simulink model "modelo_completo"  (R2023b)
settings: Solver=VariableStepAuto  StartTime=0.0  StopTime=10.0  RelTol=1e-3
undefined symbols (not defined in the file): T_hm_max, T_tm_max, tau_hm, tau_tm
settings Model: Creator=Ferran  LastModifiedBy=Ferran

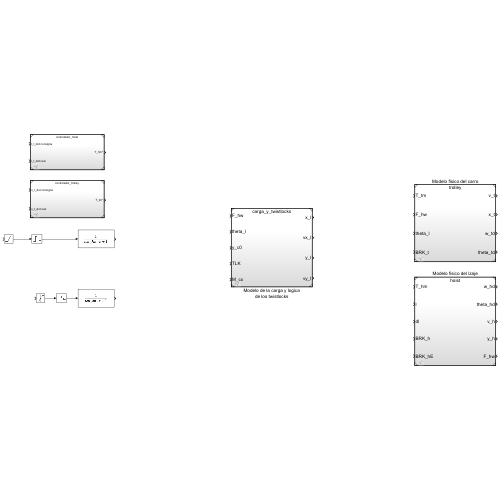
[thumbnail: Simulink's stored preview of the top-level diagram]
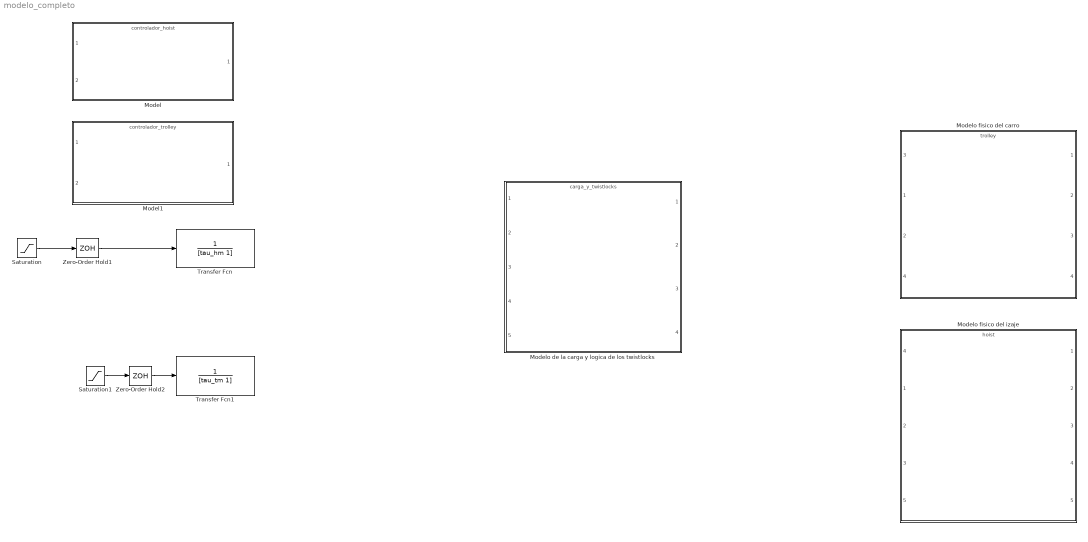
== system modelo_completo ==
  Model : ModelReference  ModelNameDialog=controlador_hoist.slx  SimulationMode=Normal  ModelReferenceVersion=2.4
  Model1 : ModelReference  ModelNameDialog=controlador_trolley.slx  SimulationMode=Normal  ModelReferenceVersion=2.1
  Modelo de la carga y logica de los twistlocks : ModelReference  ModelNameDialog=carga_y_twistlocks.slx  SimulationMode=Normal  ModelReferenceVersion=1.8
  Modelo fisico del carro : ModelReference  ModelNameDialog=trolley.slx  SimulationMode=Normal  ModelReferenceVersion=1.10
      settings: PortSchema="{\"entries\":[{\"content\":{\"sides\":[{\"content\":{\"connectorIds\":[\"In3\",\"In1\",\"In2\",\"In4\"]},\"type\":\"ConnectorPlacement.EquallySpacedRectSide\",\"uuid\":\"38a31379-7a02-4531-af9b-82f32436a2ed\"},{\"content\":{\"connectorIds\":[\"Out1\",\"Out2\",\"Out3\",\"Out4\"],\"side\":\"RIGHT\"},\"type\":\"ConnectorPlacement.EquallySpacedRectSide\",\"uuid\":\"953f32c8-509d-4a74-a27c-0c30002e5aa6\"},{\"content\":{\"side\":\"TOP\"},\"type\":\"ConnectorPlacement.EquallySpacedRectSide\",\"uuid\":\"64fb0ed3-f874-48da-a9ca-0df566987d1c\"}]},\"type\":\"ConnectorPlacement.EquallySpacedConnector\",\"uuid\":\"ea4c7909-5c74-4284-a576-3672d22ceffd\"}],\"packageUris\":[\"http://schema.mathworks.com/mf0/Connector/R2020b\"],\"version\":\"1.0\"}"
  Modelo fisico del izaje : ModelReference  ModelNameDialog=hoist.slx  SimulationMode=Normal  ModelReferenceVersion=1.12
      settings: PortSchema="{\"entries\":[{\"content\":{\"sides\":[{\"content\":{\"connectorIds\":[\"In4\",\"In1\",\"In2\",\"In3\",\"In5\"]},\"type\":\"ConnectorPlacement.EquallySpacedRectSide\",\"uuid\":\"17f6338c-3c51-40de-9973-080572c91603\"},{\"content\":{\"connectorIds\":[\"Out1\",\"Out2\",\"Out3\",\"Out4\",\"Out5\"],\"side\":\"RIGHT\"},\"type\":\"ConnectorPlacement.EquallySpacedRectSide\",\"uuid\":\"7e968b16-4cea-43bb-a5ca-e4df3289f40a\"},{\"content\":{\"side\":\"TOP\"},\"type\":\"ConnectorPlacement.EquallySpacedRectSide\",\"uuid\":\"93c8c357-b571-41b6-8c5b-1c91e217cb64\"}]},\"type\":\"ConnectorPlacement.EquallySpacedConnector\",\"uuid\":\"e66d9c43-4482-4d93-9c83-496ca9c2d477\"}],\"packageUris\":[\"http://schema.mathworks.com/mf0/Connector/R2020b\"],\"version\":\"1.0\"}"
  Saturation : Saturate  UpperLimit=T_hm_max  LowerLimit=-T_hm_max
  Saturation1 : Saturate  UpperLimit=T_tm_max  LowerLimit=-T_tm_max
  Transfer Fcn : TransferFcn  Denominator=[tau_hm 1]
  Transfer Fcn1 : TransferFcn  Denominator=[tau_tm 1]
  Zero-Order Hold1 : ZeroOrderHold  SampleTime=tau_hm
  Zero-Order Hold2 : ZeroOrderHold  SampleTime=tau_tm
  wires:
  Zero-Order Hold2/1 -> Transfer Fcn1/1
  Saturation/1 -> Zero-Order Hold1/1
  Saturation1/1 -> Zero-Order Hold2/1
  Zero-Order Hold1/1 -> Transfer Fcn/1
